simulink library "pne_pne3d_generic_std"  (R2016a)
settings: Solver=VariableStepAuto  StartTime=0.0  StopTime=10.0  RelTol=1e-3
undefined symbols (not defined in the file): sMP
(part 1 of 7)
settings Model: Creator=CAB  LastModifiedBy=CAB
settings GRTTargetCC: GeneratePreprocessorConditionals=Use local settings

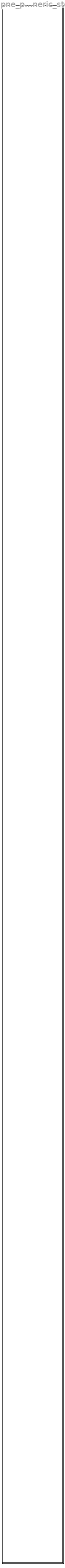
== system pne_pne3d_generic_std ==
  pne_pne3d_generic_std : Subsystem  mask{s1=sMP.phys.pne.settings_iMode, s2=sMP.phys.pne.settings_dt, initCmd='Parameters_pne_pne3d_generic_std_sf', p1=sMP.phys.pne.susp1.dxMax, p2=sMP.phys.pne.susp1.dxMin, p3=sMP.phys.pne.susp1.dxRef, p4=sMP.phys.pne.susp1.vLift, p5=sMP.phys.pne.susp1.vLow, p6=sMP.phys.pne.susp2.dxMax, p7=sMP.phys.pne.susp2.dxMin, p8=sMP.phys.pne.susp2.dxRef, p9=sMP.phys.pne.susp2.vLift, p10=sMP.phys.pne.susp2.vLow, p11=sMP.phys.pne.susp3.dxMax, p12=sMP.phys.pne.susp3.dxMin, p13=sMP.phys.pne.susp3.dxRef, p14=sMP.phys.pne.susp3.vLift, p15=sMP.phys.pne.susp3.vLow, p16=sMP.phys.pne.susp4.dxMax, p17=sMP.phys.pne.susp4.dxMin, p18=sMP.phys.pne.susp4.dxRef, p19=sMP.phys.pne.susp4.vLift, p20=sMP.phys.pne.susp4.vLow, p21=sMP.phys.pne.brk1.brakeType, p22=sMP.phys.pne.brk1.bt_A_norm, p23=sMP.phys.pne.brk1.bt_A_pad, p24=sMP.phys.pne.brk1.bt_alpha_conv_fac_cool, p25=sMP.phys.pne.brk1.bt_alpha_conv_fac_fric, p26=sMP.phys.pne.brk1.bt_base_conduction_corr, p27=sMP.phys.pne.brk1.bt_delta_r, p28=sMP.phys.pne.brk1.bt_density_correction, p29=sMP.phys.pne.brk1.bt_epsilon_corr, p30=sMP.phys.pne.brk1.bt_rad_offset, p31=sMP.phys.pne.brk1.bt_radiation_area_corr, p32=sMP.phys.pne.brk1.considerTg, p33=sMP.phys.pne.brk1.Cs, p34=sMP.phys.pne.brk1.eta, p35=sMP.phys.pne.brk1.fac_T_Dim, p36=sMP.phys.pne.brk1.fac_v_Dim, p37=sMP.phys.pne.brk1.Fdx_Dim, p38=sMP.phys.pne.brk1.Gwear, p39=sMP.phys.pne.brk1.i_Dim, p40=sMP.phys.pne.brk1.reff, p41=sMP.phys.pne.brk1.sPad_sum0, p42=sMP.phys.pne.brk1.useVarTempCalc, p43=sMP.phys.pne.brk1.wearRate_T_Dim, p44=sMP.phys.pne.brk2.brakeType, p45=sMP.phys.pne.brk2.bt_A_norm, p46=sMP.phys.pne.brk2.bt_A_pad, p47=sMP.phys.pne.brk2.bt_alpha_conv_fac_cool, p48=sMP.phys.pne.brk2.bt_alpha_conv_fac_fric, p49=sMP.phys.pne.brk2.bt_base_conduction_corr, p50=sMP.phys.pne.brk2.bt_delta_r, p51=sMP.phys.pne.brk2.bt_density_correction, p52=sMP.phys.pne.brk2.bt_epsilon_corr, p53=sMP.phys.pne.brk2.bt_rad_offset, p54=sMP.phys.pne.brk2.bt_radiation_area_corr, p55=sMP.phys.pne.brk2.considerTg, p56=sMP.phys.pne.brk2.Cs, p57=sMP.phys.pne.brk2.eta, p58=sMP.phys.pne.brk2.fac_T_Dim, p59=sMP.phys.pne.brk2.fac_v_Dim, p60=sMP.phys.pne.brk2.Fdx_Dim, p61=sMP.phys.pne.brk2.Gwear, p62=sMP.phys.pne.brk2.i_Dim, p63=sMP.phys.pne.brk2.reff, p64=sMP.phys.pne.brk2.sPad_sum0, p65=sMP.phys.pne.brk2.useVarTempCalc, p66=sMP.phys.pne.brk2.wearRate_T_Dim, p67=sMP.phys.pne.brk3.brakeType, p68=sMP.phys.pne.brk3.bt_A_norm, p69=sMP.phys.pne.brk3.bt_A_pad, p70=sMP.phys.pne.brk3.bt_alpha_conv_fac_cool, p71=sMP.phys.pne.brk3.bt_alpha_conv_fac_fric, p72=sMP.phys.pne.brk3.bt_base_conduction_corr, p73=sMP.phys.pne.brk3.bt_delta_r, p74=sMP.phys.pne.brk3.bt_density_correction, p75=sMP.phys.pne.brk3.bt_epsilon_corr, p76=sMP.phys.pne.brk3.bt_rad_offset, p77=sMP.phys.pne.brk3.bt_radiation_area_corr, p78=sMP.phys.pne.brk3.considerTg, p79=sMP.phys.pne.brk3.Cs, p80=sMP.phys.pne.brk3.eta, p81=sMP.phys.pne.brk3.fac_T_Dim, p82=sMP.phys.pne.brk3.fac_v_Dim, p83=sMP.phys.pne.brk3.Fdx_Dim, p84=sMP.phys.pne.brk3.Gwear, p85=sMP.phys.pne.brk3.i_Dim, p86=sMP.phys.pne.brk3.reff, p87=sMP.phys.pne.brk3.sPad_sum0, p88=sMP.phys.pne.brk3.useVarTempCalc, p89=sMP.phys.pne.brk3.wearRate_T_Dim, p90=sMP.phys.pne.brk4.brakeType, p91=sMP.phys.pne.brk4.bt_A_norm, p92=sMP.phys.pne.brk4.bt_A_pad, p93=sMP.phys.pne.brk4.bt_alpha_conv_fac_cool, p94=sMP.phys.pne.brk4.bt_alpha_conv_fac_fric, p95=sMP.phys.pne.brk4.bt_base_conduction_corr, p96=sMP.phys.pne.brk4.bt_delta_r, p97=sMP.phys.pne.brk4.bt_density_correction, p98=sMP.phys.pne.brk4.bt_epsilon_corr, p99=sMP.phys.pne.brk4.bt_rad_offset, p100=sMP.phys.pne.brk4.bt_radiation_area_corr, p101=sMP.phys.pne.brk4.considerTg, p102=sMP.phys.pne.brk4.Cs, p103=sMP.phys.pne.brk4.eta, p104=sMP.phys.pne.brk4.fac_T_Dim, p105=sMP.phys.pne.brk4.fac_v_Dim, p106=sMP.phys.pne.brk4.Fdx_Dim, p107=sMP.phys.pne.brk4.Gwear, p108=sMP.phys.pne.brk4.i_Dim, p109=sMP.phys.pne.brk4.reff, p110=sMP.phys.pne.brk4.sPad_sum0, p111=sMP.phys.pne.brk4.useVarTempCalc, p112=sMP.phys.pne.brk4.wearRate_T_Dim, p113=sMP.phys.pne.cyl1.dxFSpring_Dim, p114=sMP.phys.pne.cyl1.dxVolPB_Dim, p115=sMP.phys.pne.cyl1.dxVolSB_Dim, p116=sMP.phys.pne.cyl1.FNom, p117=sMP.phys.pne.cyl1.maxStroke, p118=sMP.phys.pne.cyl1.pApp, p119=sMP.phys.pne.cyl1.pNom, p120=sMP.phys.pne.cyl1.pR_PB, p121=sMP.phys.pne.cyl1.xR_PB, p122=sMP.phys.pne.cyl2.dxFSpring_Dim, p123=sMP.phys.pne.cyl2.dxVolPB_Dim, p124=sMP.phys.pne.cyl2.dxVolSB_Dim, p125=sMP.phys.pne.cyl2.FNom, p126=sMP.phys.pne.cyl2.maxStroke, p127=sMP.phys.pne.cyl2.pApp, p128=sMP.phys.pne.cyl2.pNom, p129=sMP.phys.pne.cyl2.pR_PB, p130=sMP.phys.pne.cyl2.xR_PB, p131=sMP.phys.pne.cyl3.dxFSpring_Dim, p132=sMP.phys.pne.cyl3.dxVolPB_Dim, p133=sMP.phys.pne.cyl3.dxVolSB_Dim, p134=sMP.phys.pne.cyl3.FNom, p135=sMP.phys.pne.cyl3.maxStroke, p136=sMP.phys.pne.cyl3.pApp, p137=sMP.phys.pne.cyl3.pNom, p138=sMP.phys.pne.cyl3.pR_PB, p139=sMP.phys.pne.cyl3.xR_PB, p140=sMP.phys.pne.cyl4.dxFSpring_Dim, p141=sMP.phys.pne.cyl4.dxVolPB_Dim, p142=sMP.phys.pne.cyl4.dxVolSB_Dim, p143=sMP.phys.pne.cyl4.FNom, p144=sMP.phys.pne.cyl4.maxStroke, p145=sMP.phys.pne.cyl4.pApp, p146=sMP.phys.pne.cyl4.pNom, p147=sMP.phys.pne.cyl4.pR_PB, p148=sMP.phys.pne.cyl4.xR_PB, p149=sMP.phys.pne.cylTrailer1.dxFSpring_Dim, p150=sMP.phys.pne.cylTrailer1.dxVolPB_Dim, p151=sMP.phys.pne.cylTrailer1.dxVolSB_Dim, p152=sMP.phys.pne.cylTrailer1.FNom, p153=sMP.phys.pne.cylTrailer1.maxStroke, p154=sMP.phys.pne.cylTrailer1.pApp, p155=sMP.phys.pne.cylTrailer1.pNom, p156=sMP.phys.pne.cylTrailer1.pR_PB, p157=sMP.phys.pne.cylTrailer1.xR_PB, p158=sMP.phys.pne.cylTrailer2.dxFSpring_Dim, p159=sMP.phys.pne.cylTrailer2.dxVolPB_Dim, p160=sMP.phys.pne.cylTrailer2.dxVolSB_Dim, p161=sMP.phys.pne.cylTrailer2.FNom, p162=sMP.phys.pne.cylTrailer2.maxStroke, p163=sMP.phys.pne.cylTrailer2.pApp, p164=sMP.phys.pne.cylTrailer2.pNom, p165=sMP.phys.pne.cylTrailer2.pR_PB, p166=sMP.phys.pne.cylTrailer2.xR_PB, p167=sMP.phys.pne.cylTrailer3.dxFSpring_Dim, p168=sMP.phys.pne.cylTrailer3.dxVolPB_Dim, p169=sMP.phys.pne.cylTrailer3.dxVolSB_Dim, p170=sMP.phys.pne.cylTrailer3.FNom, p171=sMP.phys.pne.cylTrailer3.maxStroke, p172=sMP.phys.pne.cylTrailer3.pApp, p173=sMP.phys.pne.cylTrailer3.pNom, p174=sMP.phys.pne.cylTrailer3.pR_PB, p175=sMP.phys.pne.cylTrailer3.xR_PB, p176=sMP.phys.pne.brkTrailer1.brakeType, p177=sMP.phys.pne.brkTrailer1.bt_A_norm, p178=sMP.phys.pne.brkTrailer1.bt_A_pad, p179=sMP.phys.pne.brkTrailer1.bt_alpha_conv_fac_cool, p180=sMP.phys.pne.brkTrailer1.bt_alpha_conv_fac_fric, p181=sMP.phys.pne.brkTrailer1.bt_base_conduction_corr, p182=sMP.phys.pne.brkTrailer1.bt_delta_r, p183=sMP.phys.pne.brkTrailer1.bt_density_correction, p184=sMP.phys.pne.brkTrailer1.bt_epsilon_corr, p185=sMP.phys.pne.brkTrailer1.bt_rad_offset, p186=sMP.phys.pne.brkTrailer1.bt_radiation_area_corr, p187=sMP.phys.pne.brkTrailer1.considerTg, p188=sMP.phys.pne.brkTrailer1.Cs, p189=sMP.phys.pne.brkTrailer1.eta, p190=sMP.phys.pne.brkTrailer1.fac_T_Dim, p191=sMP.phys.pne.brkTrailer1.fac_v_Dim, p192=sMP.phys.pne.brkTrailer1.Fdx_Dim, p193=sMP.phys.pne.brkTrailer1.Gwear, p194=sMP.phys.pne.brkTrailer1.i_Dim, p195=sMP.phys.pne.brkTrailer1.reff, p196=sMP.phys.pne.brkTrailer1.sPad_sum0, p197=sMP.phys.pne.brkTrailer1.useVarTempCalc, p198=sMP.phys.pne.brkTrailer1.wearRate_T_Dim, p199=sMP.phys.pne.brkTrailer2.brakeType, p200=sMP.phys.pne.brkTrailer2.bt_A_norm, p201=sMP.phys.pne.brkTrailer2.bt_A_pad, p202=sMP.phys.pne.brkTrailer2.bt_alpha_conv_fac_cool, p203=sMP.phys.pne.brkTrailer2.bt_alpha_conv_fac_fric, p204=sMP.phys.pne.brkTrailer2.bt_base_conduction_corr, p205=sMP.phys.pne.brkTrailer2.bt_delta_r, p206=sMP.phys.pne.brkTrailer2.bt_density_correction, p207=sMP.phys.pne.brkTrailer2.bt_epsilon_corr, p208=sMP.phys.pne.brkTrailer2.bt_rad_offset, p209=sMP.phys.pne.brkTrailer2.bt_radiation_area_corr, p210=sMP.phys.pne.brkTrailer2.considerTg, p211=sMP.phys.pne.brkTrailer2.Cs, p212=sMP.phys.pne.brkTrailer2.eta, p213=sMP.phys.pne.brkTrailer2.fac_T_Dim, p214=sMP.phys.pne.brkTrailer2.fac_v_Dim, p215=sMP.phys.pne.brkTrailer2.Fdx_Dim, p216=sMP.phys.pne.brkTrailer2.Gwear, p217=sMP.phys.pne.brkTrailer2.i_Dim, p218=sMP.phys.pne.brkTrailer2.reff, p219=sMP.phys.pne.brkTrailer2.sPad_sum0, p220=sMP.phys.pne.brkTrailer2.useVarTempCalc, p221=sMP.phys.pne.brkTrailer2.wearRate_T_Dim, p222=sMP.phys.pne.brkTrailer3.brakeType, p223=sMP.phys.pne.brkTrailer3.bt_A_norm, p224=sMP.phys.pne.brkTrailer3.bt_A_pad, p225=sMP.phys.pne.brkTrailer3.bt_alpha_conv_fac_cool, p226=sMP.phys.pne.brkTrailer3.bt_alpha_conv_fac_fric, p227=sMP.phys.pne.brkTrailer3.bt_base_conduction_corr, p228=sMP.phys.pne.brkTrailer3.bt_delta_r, p229=sMP.phys.pne.brkTrailer3.bt_density_correction, p230=sMP.phys.pne.brkTrailer3.bt_epsilon_corr, p231=sMP.phys.pne.brkTrailer3.bt_rad_offset, p232=sMP.phys.pne.brkTrailer3.bt_radiation_area_corr, p233=sMP.phys.pne.brkTrailer3.considerTg, p234=sMP.phys.pne.brkTrailer3.Cs, p235=sMP.phys.pne.brkTrailer3.eta, p236=sMP.phys.pne.brkTrailer3.fac_T_Dim, p237=sMP.phys.pne.brkTrailer3.fac_v_Dim, p238=sMP.phys.pne.brkTrailer3.Fdx_Dim, p239=sMP.phys.pne.brkTrailer3.Gwear, p240=sMP.phys.pne.brkTrailer3.i_Dim, p241=sMP.phys.pne.brkTrailer3.reff, p242=sMP.phys.pne.brkTrailer3.sPad_sum0, p243=sMP.phys.pne.brkTrailer3.useVarTempCalc, p244=sMP.phys.pne.brkTrailer3.wearRate_T_Dim, p245=sMP.phys.pne.circ.T_pipe_AM_ABSValve_FL, p246=sMP.phys.pne.circ.T_pipe_AM_ABSValve_FR, p247=sMP.phys.pne.circ.T_pipe_AM_BC_AL, p248=sMP.phys.pne.circ.T_pipe_AM_BC_AR, p249=sMP.phys.pne.circ.T_pipe_AM_BC_RL, p250=sMP.phys.pne.circ.T_pipe_AM_BC_RR, p251=sMP.phys.pne.circTrlr.flagTrailerABS, p252=sMP.phys.pne.circTrlr.T_pipe_Trailer_RV_Front, p253=sMP.phys.pne.circTrlr.T_pipe_Trailer_RV_Front_Rear, p254=sMP.phys.pne.circTrlr.VTrailer, p255=sMP.phys.pne.com.pACoverflow, p256=sMP.phys.pne.auxil.Drs_dVClose, p257=sMP.phys.pne.auxil.Drs_dVOpen, p258=sMP.phys.pne.auxil.Drs_pMeas, p259=sMP.phys.pne.auxil.Drs_tClose, p260=sMP.phys.pne.auxil.Drs_tOpen, p261=sMP.phys.pne.in.ebs_AdditionalAxle_left_pDmd, p262=sMP.phys.pne.in.ebs_AdditionalAxle_left_setABS, p263=sMP.phys.pne.in.ebs_AdditionalAxle_right_pDmd, p264=sMP.phys.pne.in.ebs_AdditionalAxle_right_setABS, p265=sMP.phys.pne.in.ebs_ESCsens_y_acceleration, p266=sMP.phys.pne.in.ebs_FrontAxle_left_pDmd, p267=sMP.phys.pne.in.ebs_FrontAxle_left_setABS, p268=sMP.phys.pne.in.ebs_FrontAxle_right_pDmd, p269=sMP.phys.pne.in.ebs_FrontAxle_right_setABS, p270=sMP.phys.pne.in.ebs_RearAxle_left_pDmd, p271=sMP.phys.pne.in.ebs_RearAxle_left_setABS, p272=sMP.phys.pne.in.ebs_RearAxle_right_pDmd, p273=sMP.phys.pne.in.ebs_RearAxle_right_setABS, p274=sMP.phys.pne.in.ebs_sBSP_stABSInValve_Addl_Left, p275=sMP.phys.pne.in.ebs_sBSP_stABSInValve_Addl_Right, p276=sMP.phys.pne.in.ebs_sBSP_stABSInValve_Front_Left, p277=sMP.phys.pne.in.ebs_sBSP_stABSInValve_Front_Right, p278=sMP.phys.pne.in.ebs_sBSP_stABSInValve_RCMax_Front, p279=sMP.phys.pne.in.ebs_sBSP_stABSInValve_RCMax_Rear, p280=sMP.phys.pne.in.ebs_sBSP_stABSInValve_Rear_Left, p281=sMP.phys.pne.in.ebs_sBSP_stABSInValve_Rear_Right, p282=sMP.phys.pne.in.ebs_sBSP_stABSOutValve_Addl_Left, p283=sMP.phys.pne.in.ebs_sBSP_stABSOutValve_Addl_Right, p284=sMP.phys.pne.in.ebs_sBSP_stABSOutValve_Front_Left, p285=sMP.phys.pne.in.ebs_sBSP_stABSOutValve_Front_Right, p286=sMP.phys.pne.in.ebs_sBSP_stABSOutValve_RCMax_Front, p287=sMP.phys.pne.in.ebs_sBSP_stABSOutValve_RCMax_Rear, p288=sMP.phys.pne.in.ebs_sBSP_stABSOutValve_Rear_Left, p289=sMP.phys.pne.in.ebs_sBSP_stABSOutValve_Rear_Right, p290=sMP.phys.pne.in.ebs_sBSP_stAPCVBuValve, p291=sMP.phys.pne.in.ebs_sBSP_stAPCVInValve, p292=sMP.phys.pne.in.ebs_sBSP_stAPCVOutValve, p293=sMP.phys.pne.in.ebs_sBSP_stAtcCutOffValve, p294=sMP.phys.pne.in.ebs_sBSP_stAxmoBuValve, p295=sMP.phys.pne.in.ebs_sBSP_stAxmoInValve_Rear_Left, p296=sMP.phys.pne.in.ebs_sBSP_stAxmoInValve_Rear_Right, p297=sMP.phys.pne.in.ebs_sBSP_stAxmoOutValve_Rear_Left, p298=sMP.phys.pne.in.ebs_sBSP_stAxmoOutValve_Rear_Right, p299=sMP.phys.pne.in.ebs_sBSP_stCMaxBuValve, p300=sMP.phys.pne.in.ebs_sBSP_stCMaxInValve_Rear_Left, p301=sMP.phys.pne.in.ebs_sBSP_stCMaxInValve_Rear_Right, p302=sMP.phys.pne.in.ebs_sBSP_stCMaxOutValve_Rear_Left, p303=sMP.phys.pne.in.ebs_sBSP_stCMaxOutValve_Rear_Right, p304=sMP.phys.pne.in.ebs_sBSP_stRCMaxInValve_Front, p305=sMP.phys.pne.in.ebs_sBSP_stRCMaxInValve_Rear, p306=sMP.phys.pne.in.ebs_sBSP_stRCMaxOutValve_Front, p307=sMP.phys.pne.in.ebs_sBSP_stRCMaxOutValve_Rear, p308=sMP.phys.pne.in.ebs_sBSP_stTCVBuValve, p309=sMP.phys.pne.in.ebs_sBSP_stTCVInValve, p310=sMP.phys.pne.in.ebs_sBSP_stTCVOutValve, p311=sMP.phys.pne.in.ebs_sil_AAle_force, p312=sMP.phys.pne.in.ebs_sil_AAle_vel, p313=sMP.phys.pne.in.ebs_sil_AAri_force, p314=sMP.phys.pne.in.ebs_sil_AAri_vel, p315=sMP.phys.pne.in.ebs_sil_FAle_force, p316=sMP.phys.pne.in.ebs_sil_FAle_vel, p317=sMP.phys.pne.in.ebs_sil_FAri_force, p318=sMP.phys.pne.in.ebs_sil_FAri_vel, p319=sMP.phys.pne.in.ebs_sil_RAle_force, p320=sMP.phys.pne.in.ebs_sil_RAle_vel, p321=sMP.phys.pne.in.ebs_sil_RAri_force, p322=sMP.phys.pne.in.ebs_sil_RAri_vel, p323=sMP.phys.pne.in.ebs_st3by2_First, p324=sMP.phys.pne.in.ebs_st3by2_Second, p325=sMP.phys.pne.in.ebs_TCV_pDmd, p326=sMP.phys.pne.in.env_air_frontVel, p327=sMP.phys.pne.in.env_pressure, p328=sMP.phys.pne.in.env_Temperature, p329=sMP.phys.pne.in.Failure_electric_circuit_AA, p330=sMP.phys.pne.in.Failure_electric_circuit_FA, p331=sMP.phys.pne.in.Failure_electric_circuit_RA, p332=sMP.phys.pne.in.Failure_pneumatic_circuit_FA, p333=sMP.phys.pne.in.Failure_pneumatic_circuit_RA, p334=sMP.phys.pne.out.pne_AirConsumptionFlow_AirSuspension, p335=sMP.phys.pne.out.pne_AirConsumptionFlow_auxiliaries, p336=sMP.phys.pne.out.pne_AirConsumptionFlow_doors, p337=sMP.phys.pne.out.pne_AirConsumptionFlow_EnduranceBrakes, p338=sMP.phys.pne.out.pne_AirConsumptionFlow_engine, p339=sMP.phys.pne.out.pne_AirConsumptionFlow_gearbox, p340=sMP.phys.pne.out.pne_AirConsumptionFlow_leakage, p341=sMP.phys.pne.out.pne_AirConsumptionFlow_PowerBoost, p342=sMP.phys.pne.out.pne_AirConsumptionFlow_SCR, p343=sMP.phys.pne.out.pne_brk_Actual_Pressure_AL, p344=sMP.phys.pne.out.pne_brk_Actual_Pressure_AR, p345=sMP.phys.pne.out.pne_brk_Actual_Pressure_FA, p346=sMP.phys.pne.out.pne_brk_Actual_Pressure_FOPB, p347=sMP.phys.pne.out.pne_brk_Actual_Pressure_Front, p348=sMP.phys.pne.out.pne_brk_Actual_Pressure_Rear, p349=sMP.phys.pne.out.pne_brk_Actual_Pressure_RL, p350=sMP.phys.pne.out.pne_brk_Actual_Pressure_RR, p351=sMP.phys.pne.out.pne_brk_Actual_Pressure_TCV, p352=sMP.phys.pne.out.pne_brk_AdditionalAxle_AxMo_left_rotVel, p353=sMP.phys.pne.out.pne_brk_AdditionalAxle_AxMo_right_rotVel, p354=sMP.phys.pne.out.pne_brk_AdditionalAxle_left_pAct, p355=sMP.phys.pne.out.pne_brk_AdditionalAxle_left_rotVel, p356=sMP.phys.pne.out.pne_brk_AdditionalAxle_right_pAct, p357=sMP.phys.pne.out.pne_brk_AdditionalAxle_right_rotVel, p358=sMP.phys.pne.in.pne_brk_AirCompressor_angAcc, p359=sMP.phys.pne.in.pne_brk_AirCompressor_angPos, p360=sMP.phys.pne.in.pne_brk_AirCompressor_angVel, p361=sMP.phys.pne.out.pne_brk_AirCompressor_delivery, p362=sMP.phys.pne.out.pne_brk_AirCompressor_torque, p363=sMP.phys.pne.out.pne_brk_AirConsumpEng_massfracH2O, p364=sMP.phys.pne.in.pne_brk_AirConsumpEng_mdot, p365=sMP.phys.pne.out.pne_brk_AirConsumpEng_pressure, p366=sMP.phys.pne.out.pne_brk_AirConsumpEng_Temperature, p367=sMP.phys.pne.out.pne_brk_AirConsumpRet_massfracH2O, p368=sMP.phys.pne.in.pne_brk_AirConsumpRet_mdot, p369=sMP.phys.pne.out.pne_brk_AirConsumpRet_pressure, p370=sMP.phys.pne.out.pne_brk_AirConsumpRet_Temperature, p371=sMP.phys.pne.out.pne_brk_AirConsumpTx_massfracH2O, p372=sMP.phys.pne.in.pne_brk_AirConsumpTx_mdot, p373=sMP.phys.pne.out.pne_brk_AirConsumpTx_pressure, p374=sMP.phys.pne.out.pne_brk_AirConsumpTx_Temperature, p375=sMP.phys.pne.out.pne_brk_Axle1_BrakingForce_at8p5bar, p376=sMP.phys.pne.out.pne_brk_Axle1_BrakingPower, p377=sMP.phys.pne.in.pne_brk_Axle1_left_angAcc, p378=sMP.phys.pne.in.pne_brk_Axle1_left_angPos, p379=sMP.phys.pne.in.pne_brk_Axle1_left_angVel, p380=sMP.phys.pne.out.pne_brk_Axle1_left_kvT, p381=sMP.phys.pne.out.pne_brk_Axle1_left_sPad_sum, p382=sMP.phys.pne.out.pne_brk_Axle1_left_Tcooldown, p383=sMP.phys.pne.out.pne_brk_Axle1_left_Tfriction, p384=sMP.phys.pne.out.pne_brk_Axle1_left_Tinterior, p385=sMP.phys.pne.out.pne_brk_Axle1_left_torque, p386=sMP.phys.pne.out.pne_brk_Axle1_left_torque_grinding, p387=sMP.phys.pne.in.pne_brk_Axle1_right_angAcc, p388=sMP.phys.pne.in.pne_brk_Axle1_right_angPos, p389=sMP.phys.pne.in.pne_brk_Axle1_right_angVel, p390=sMP.phys.pne.out.pne_brk_Axle1_right_kvT, p391=sMP.phys.pne.out.pne_brk_Axle1_right_sPad_sum, p392=sMP.phys.pne.out.pne_brk_Axle1_right_Tcooldown, p393=sMP.phys.pne.out.pne_brk_Axle1_right_Tfriction, p394=sMP.phys.pne.out.pne_brk_Axle1_right_Tinterior, p395=sMP.phys.pne.out.pne_brk_Axle1_right_torque, p396=sMP.phys.pne.out.pne_brk_Axle1_right_torque_grinding, p397=sMP.phys.pne.out.pne_brk_Axle1_torque_sns, p398=sMP.phys.pne.out.pne_brk_Axle1Brake_Fcyl, p399=sMP.phys.pne.out.pne_brk_Axle1Brake_left_pRel, p400=sMP.phys.pne.out.pne_brk_Axle1Brake_right_pRel, p401=sMP.phys.pne.out.pne_brk_Axle1Brake_stroke, p402=sMP.phys.pne.out.pne_brk_Axle1Brake_Vol, p403=sMP.phys.pne.out.pne_brk_Axle2_BrakingForce_at8p5bar, p404=sMP.phys.pne.out.pne_brk_Axle2_BrakingPower, p405=sMP.phys.pne.in.pne_brk_Axle2_left_angAcc, p406=sMP.phys.pne.in.pne_brk_Axle2_left_angPos, p407=sMP.phys.pne.in.pne_brk_Axle2_left_angVel, p408=sMP.phys.pne.out.pne_brk_Axle2_left_kvT, p409=sMP.phys.pne.out.pne_brk_Axle2_left_sPad_sum, p410=sMP.phys.pne.out.pne_brk_Axle2_left_Tcooldown, p411=sMP.phys.pne.out.pne_brk_Axle2_left_Tfriction, p412=sMP.phys.pne.out.pne_brk_Axle2_left_Tinterior, p413=sMP.phys.pne.out.pne_brk_Axle2_left_torque, p414=sMP.phys.pne.out.pne_brk_Axle2_left_torque_grinding, p415=sMP.phys.pne.in.pne_brk_Axle2_right_angAcc, p416=sMP.phys.pne.in.pne_brk_Axle2_right_angPos, p417=sMP.phys.pne.in.pne_brk_Axle2_right_angVel, p418=sMP.phys.pne.out.pne_brk_Axle2_right_kvT, p419=sMP.phys.pne.out.pne_brk_Axle2_right_sPad_sum, p420=sMP.phys.pne.out.pne_brk_Axle2_right_Tcooldown, p421=sMP.phys.pne.out.pne_brk_Axle2_right_Tfriction, p422=sMP.phys.pne.out.pne_brk_Axle2_right_Tinterior, p423=sMP.phys.pne.out.pne_brk_Axle2_right_torque, p424=sMP.phys.pne.out.pne_brk_Axle2_right_torque_grinding, p425=sMP.phys.pne.out.pne_brk_Axle2_torque_sns, p426=sMP.phys.pne.out.pne_brk_Axle2Brake_Fcyl, p427=sMP.phys.pne.out.pne_brk_Axle2Brake_left_pRel, p428=sMP.phys.pne.out.pne_brk_Axle2Brake_right_pRel, p429=sMP.phys.pne.out.pne_brk_Axle2Brake_stroke, p430=sMP.phys.pne.out.pne_brk_Axle2Brake_Vol, p431=sMP.phys.pne.out.pne_brk_Axle3_BrakingForce_at8p5bar, p432=sMP.phys.pne.out.pne_brk_Axle3_BrakingPower, p433=sMP.phys.pne.in.pne_brk_Axle3_left_angAcc, p434=sMP.phys.pne.in.pne_brk_Axle3_left_angPos, p435=sMP.phys.pne.in.pne_brk_Axle3_left_angVel, p436=sMP.phys.pne.out.pne_brk_Axle3_left_kvT, p437=sMP.phys.pne.out.pne_brk_Axle3_left_sPad_sum, p438=sMP.phys.pne.out.pne_brk_Axle3_left_Tcooldown, p439=sMP.phys.pne.out.pne_brk_Axle3_left_Tfriction, p440=sMP.phys.pne.out.pne_brk_Axle3_left_Tinterior, p441=sMP.phys.pne.out.pne_brk_Axle3_left_torque, p442=sMP.phys.pne.out.pne_brk_Axle3_left_torque_grinding, p443=sMP.phys.pne.in.pne_brk_Axle3_right_angAcc, p444=sMP.phys.pne.in.pne_brk_Axle3_right_angPos, p445=sMP.phys.pne.in.pne_brk_Axle3_right_angVel, p446=sMP.phys.pne.out.pne_brk_Axle3_right_kvT, p447=sMP.phys.pne.out.pne_brk_Axle3_right_sPad_sum, p448=sMP.phys.pne.out.pne_brk_Axle3_right_Tcooldown, p449=sMP.phys.pne.out.pne_brk_Axle3_right_Tfriction, p450=sMP.phys.pne.out.pne_brk_Axle3_right_Tinterior, p451=sMP.phys.pne.out.pne_brk_Axle3_right_torque, p452=sMP.phys.pne.out.pne_brk_Axle3_right_torque_grinding, p453=sMP.phys.pne.out.pne_brk_Axle3_torque_sns, p454=sMP.phys.pne.out.pne_brk_Axle3Brake_Fcyl, p455=sMP.phys.pne.out.pne_brk_Axle3Brake_left_pRel, p456=sMP.phys.pne.out.pne_brk_Axle3Brake_right_pRel, p457=sMP.phys.pne.out.pne_brk_Axle3Brake_stroke, p458=sMP.phys.pne.out.pne_brk_Axle3Brake_Vol, p459=sMP.phys.pne.out.pne_brk_Axle4_BrakingForce_at8p5bar, p460=sMP.phys.pne.out.pne_brk_Axle4_BrakingPower, p461=sMP.phys.pne.in.pne_brk_Axle4_left_angAcc, p462=sMP.phys.pne.in.pne_brk_Axle4_left_angPos, p463=sMP.phys.pne.in.pne_brk_Axle4_left_angVel, p464=sMP.phys.pne.out.pne_brk_Axle4_left_kvT, p465=sMP.phys.pne.out.pne_brk_Axle4_left_sPad_sum, p466=sMP.phys.pne.out.pne_brk_Axle4_left_Tcooldown, p467=sMP.phys.pne.out.pne_brk_Axle4_left_Tfriction, p468=sMP.phys.pne.out.pne_brk_Axle4_left_Tinterior, p469=sMP.phys.pne.out.pne_brk_Axle4_left_torque, p470=sMP.phys.pne.out.pne_brk_Axle4_left_torque_grinding, p471=sMP.phys.pne.in.pne_brk_Axle4_right_angAcc, p472=sMP.phys.pne.in.pne_brk_Axle4_right_angPos, p473=sMP.phys.pne.in.pne_brk_Axle4_right_angVel, p474=sMP.phys.pne.out.pne_brk_Axle4_right_kvT, p475=sMP.phys.pne.out.pne_brk_Axle4_right_sPad_sum, p476=sMP.phys.pne.out.pne_brk_Axle4_right_Tcooldown, p477=sMP.phys.pne.out.pne_brk_Axle4_right_Tfriction, p478=sMP.phys.pne.out.pne_brk_Axle4_right_Tinterior, p479=sMP.phys.pne.out.pne_brk_Axle4_right_torque, p480=sMP.phys.pne.out.pne_brk_Axle4_right_torque_grinding, p481=sMP.phys.pne.out.pne_brk_Axle4_torque_sns, p482=sMP.phys.pne.out.pne_brk_Axle4Brake_Fcyl, p483=sMP.phys.pne.out.pne_brk_Axle4Brake_left_pRel, p484=sMP.phys.pne.out.pne_brk_Axle4Brake_right_pRel, p485=sMP.phys.pne.out.pne_brk_Axle4Brake_stroke, p486=sMP.phys.pne.out.pne_brk_Axle4Brake_Vol, p487=sMP.phys.pne.out.pne_brk_BrkWearAALt, p488=sMP.phys.pne.out.pne_brk_BrkWearAARt, p489=sMP.phys.pne.out.pne_brk_BrkWearFA1Lt, p490=sMP.phys.pne.out.pne_brk_BrkWearFA1Rt, p491=sMP.phys.pne.out.pne_brk_BrkWearFA2Lt, p492=sMP.phys.pne.out.pne_brk_BrkWearFA2Rt, p493=sMP.phys.pne.out.pne_brk_BrkWearRA1Lt, p494=sMP.phys.pne.out.pne_brk_BrkWearRA1Rt, p495=sMP.phys.pne.out.pne_brk_BrkWearRA2Lt, p496=sMP.phys.pne.out.pne_brk_BrkWearRA2Rt, p497=sMP.phys.pne.out.pne_brk_CompON, p498=sMP.phys.pne.out.pne_brk_CompOut_Temp, p499=sMP.phys.pne.in.pne_brk_CompressorInlet_massfracH2O, p500=sMP.phys.pne.out.pne_brk_CompressorInlet_mdot, p501=sMP.phys.pne.in.pne_brk_CompressorInlet_pressure, p502=sMP.phys.pne.in.pne_brk_CompressorInlet_Temperature, p503=sMP.phys.pne.out.pne_brk_CoolingPipe_pRel, p504=sMP.phys.pne.out.pne_brk_CoolingPipe_Temp, p505=sMP.phys.pne.out.pne_brk_EAPU_pRel, p506=sMP.phys.pne.out.pne_brk_EAPU_Temp, p507=sMP.phys.pne.out.pne_brk_FrontAxle_left_rotVel, p508=sMP.phys.pne.out.pne_brk_FrontAxle_pAct, p509=sMP.phys.pne.out.pne_brk_FrontAxle_right_rotVel, p510=sMP.phys.pne.out.pne_brk_PowerBoost_massfracH2O, p511=sMP.phys.pne.in.pne_brk_PowerBoost_mdot, p512=sMP.phys.pne.out.pne_brk_PowerBoost_pressure, p513=sMP.phys.pne.out.pne_brk_PowerBoost_Temperature, p514=sMP.phys.pne.out.pne_brk_pRelPkBrk, p515=sMP.phys.pne.out.pne_brk_RearAxle_left_pAct, p516=sMP.phys.pne.out.pne_brk_RearAxle_left_rotVel, p517=sMP.phys.pne.out.pne_brk_RearAxle_right_pAct, p518=sMP.phys.pne.out.pne_brk_RearAxle_right_rotVel, p519=sMP.phys.pne.out.pne_brk_reg_active, p520=sMP.phys.pne.out.pne_brk_rotVel_al, p521=sMP.phys.pne.out.pne_brk_rotVel_ar, p522=sMP.phys.pne.out.pne_brk_rotVel_fl, p523=sMP.phys.pne.out.pne_brk_rotVel_fr, p524=sMP.phys.pne.out.pne_brk_rotVel_rl, p525=sMP.phys.pne.out.pne_brk_rotVel_rr, p526=sMP.phys.pne.out.pne_brk_rotVel_t1l, p527=sMP.phys.pne.out.pne_brk_rotVel_t1r, p528=sMP.phys.pne.out.pne_brk_rotVel_t2l, p529=sMP.phys.pne.out.pne_brk_rotVel_t2r, p530=sMP.phys.pne.out.pne_brk_rotVel_t3l, p531=sMP.phys.pne.out.pne_brk_rotVel_t3r, p532=sMP.phys.pne.out.pne_brk_TCV_pAct, p533=sMP.phys.pne.out.pne_brk_Trailer_RV_Front_pAct, p534=sMP.phys.pne.out.pne_brk_Trailer_RV_Rear_pAct, p535=sMP.phys.pne.out.pne_brk_TrailerAxle1_BrakingForce_at8p5bar, p536=sMP.phys.pne.out.pne_brk_TrailerAxle1_BrakingPower, p537=sMP.phys.pne.in.pne_brk_TrailerAxle1_left_angAcc, p538=sMP.phys.pne.in.pne_brk_TrailerAxle1_left_angPos, p539=sMP.phys.pne.in.pne_brk_TrailerAxle1_left_angVel, p540=sMP.phys.pne.out.pne_brk_TrailerAxle1_left_kvT, p541=sMP.phys.pne.out.pne_brk_TrailerAxle1_left_sPad_sum, p542=sMP.phys.pne.out.pne_brk_TrailerAxle1_left_Tcooldown, p543=sMP.phys.pne.out.pne_brk_TrailerAxle1_left_Tfriction, p544=sMP.phys.pne.out.pne_brk_TrailerAxle1_left_Tinterior, p545=sMP.phys.pne.out.pne_brk_TrailerAxle1_left_torque, p546=sMP.phys.pne.out.pne_brk_TrailerAxle1_left_torque_grinding, p547=sMP.phys.pne.in.pne_brk_TrailerAxle1_right_angAcc, p548=sMP.phys.pne.in.pne_brk_TrailerAxle1_right_angPos, p549=sMP.phys.pne.in.pne_brk_TrailerAxle1_right_angVel, p550=sMP.phys.pne.out.pne_brk_TrailerAxle1_right_kvT, p551=sMP.phys.pne.out.pne_brk_TrailerAxle1_right_sPad_sum, p552=sMP.phys.pne.out.pne_brk_TrailerAxle1_right_Tcooldown, p553=sMP.phys.pne.out.pne_brk_TrailerAxle1_right_Tfriction, p554=sMP.phys.pne.out.pne_brk_TrailerAxle1_right_Tinterior, p555=sMP.phys.pne.out.pne_brk_TrailerAxle1_right_torque, p556=sMP.phys.pne.out.pne_brk_TrailerAxle1_right_torque_grinding, p557=sMP.phys.pne.out.pne_brk_TrailerAxle1_torque_sns, p558=sMP.phys.pne.out.pne_brk_TrailerAxle1Brake_Fcyl, p559=sMP.phys.pne.out.pne_brk_TrailerAxle1Brake_left_pRel, p560=sMP.phys.pne.out.pne_brk_TrailerAxle1Brake_right_pRel, p561=sMP.phys.pne.out.pne_brk_TrailerAxle1Brake_stroke, p562=sMP.phys.pne.out.pne_brk_TrailerAxle1Brake_Vol, p563=sMP.phys.pne.out.pne_brk_TrailerAxle2_BrakingForce_at8p5bar, p564=sMP.phys.pne.out.pne_brk_TrailerAxle2_BrakingPower, p565=sMP.phys.pne.in.pne_brk_TrailerAxle2_left_angAcc, p566=sMP.phys.pne.in.pne_brk_TrailerAxle2_left_angPos, p567=sMP.phys.pne.in.pne_brk_TrailerAxle2_left_angVel, p568=sMP.phys.pne.out.pne_brk_TrailerAxle2_left_kvT, p569=sMP.phys.pne.out.pne_brk_TrailerAxle2_left_sPad_sum, p570=sMP.phys.pne.out.pne_brk_TrailerAxle2_left_Tcooldown, p571=sMP.phys.pne.out.pne_brk_TrailerAxle2_left_Tfriction, p572=sMP.phys.pne.out.pne_brk_TrailerAxle2_left_Tinterior, p573=sMP.phys.pne.out.pne_brk_TrailerAxle2_left_torque, p574=sMP.phys.pne.out.pne_brk_TrailerAxle2_left_torque_grinding, p575=sMP.phys.pne.in.pne_brk_TrailerAxle2_right_angAcc, p576=sMP.phys.pne.in.pne_brk_TrailerAxle2_right_angPos, p577=sMP.phys.pne.in.pne_brk_TrailerAxle2_right_angVel, p578=sMP.phys.pne.out.pne_brk_TrailerAxle2_right_kvT, p579=sMP.phys.pne.out.pne_brk_TrailerAxle2_right_sPad_sum, p580=sMP.phys.pne.out.pne_brk_TrailerAxle2_right_Tcooldown, p581=sMP.phys.pne.out.pne_brk_TrailerAxle2_right_Tfriction, p582=sMP.phys.pne.out.pne_brk_TrailerAxle2_right_Tinterior, p583=sMP.phys.pne.out.pne_brk_TrailerAxle2_right_torque, p584=sMP.phys.pne.out.pne_brk_TrailerAxle2_right_torque_grinding, p585=sMP.phys.pne.out.pne_brk_TrailerAxle2_torque_sns, p586=sMP.phys.pne.out.pne_brk_TrailerAxle2Brake_Fcyl, p587=sMP.phys.pne.out.pne_brk_TrailerAxle2Brake_left_pRel, p588=sMP.phys.pne.out.pne_brk_TrailerAxle2Brake_right_pRel, p589=sMP.phys.pne.out.pne_brk_TrailerAxle2Brake_stroke, p590=sMP.phys.pne.out.pne_brk_TrailerAxle2Brake_Vol, p591=sMP.phys.pne.out.pne_brk_TrailerAxle3_BrakingForce_at8p5bar, p592=sMP.phys.pne.out.pne_brk_TrailerAxle3_BrakingPower, p593=sMP.phys.pne.in.pne_brk_TrailerAxle3_left_angAcc, p594=sMP.phys.pne.in.pne_brk_TrailerAxle3_left_angPos, p595=sMP.phys.pne.in.pne_brk_TrailerAxle3_left_angVel, p596=sMP.phys.pne.out.pne_brk_TrailerAxle3_left_kvT, p597=sMP.phys.pne.out.pne_brk_TrailerAxle3_left_sPad_sum, p598=sMP.phys.pne.out.pne_brk_TrailerAxle3_left_Tcooldown, p599=sMP.phys.pne.out.pne_brk_TrailerAxle3_left_Tfriction, p600=sMP.phys.pne.out.pne_brk_TrailerAxle3_left_Tinterior, p601=sMP.phys.pne.out.pne_brk_TrailerAxle3_left_torque, p602=sMP.phys.pne.out.pne_brk_TrailerAxle3_left_torque_grinding, p603=sMP.phys.pne.in.pne_brk_TrailerAxle3_right_angAcc, p604=sMP.phys.pne.in.pne_brk_TrailerAxle3_right_angPos, p605=sMP.phys.pne.in.pne_brk_TrailerAxle3_right_angVel, p606=sMP.phys.pne.out.pne_brk_TrailerAxle3_right_kvT, p607=sMP.phys.pne.out.pne_brk_TrailerAxle3_right_sPad_sum, p608=sMP.phys.pne.out.pne_brk_TrailerAxle3_right_Tcooldown, p609=sMP.phys.pne.out.pne_brk_TrailerAxle3_right_Tfriction, p610=sMP.phys.pne.out.pne_brk_TrailerAxle3_right_Tinterior, p611=sMP.phys.pne.out.pne_brk_TrailerAxle3_right_torque, p612=sMP.phys.pne.out.pne_brk_TrailerAxle3_right_torque_grinding, p613=sMP.phys.pne.out.pne_brk_TrailerAxle3_torque_sns, p614=sMP.phys.pne.out.pne_brk_TrailerAxle3Brake_Fcyl, p615=sMP.phys.pne.out.pne_brk_TrailerAxle3Brake_left_pRel, p616=sMP.phys.pne.out.pne_brk_TrailerAxle3Brake_right_pRel, p617=sMP.phys.pne.out.pne_brk_TrailerAxle3Brake_stroke, p618=sMP.phys.pne.out.pne_brk_TrailerAxle3Brake_Vol, p619=sMP.phys.pne.out.pne_brk_V1_pRel, p620=sMP.phys.pne.out.pne_brk_V1_Temp, p621=sMP.phys.pne.out.pne_brk_V2_pRel, p622=sMP.phys.pne.out.pne_brk_V2_Temp, p623=sMP.phys.pne.out.pne_brk_V3_pRel, p624=sMP.phys.pne.out.pne_brk_V3_Temp, p625=sMP.phys.pne.out.pne_brk_V4_pRel, p626=sMP.phys.pne.out.pne_brk_V4_Temp, p627=sMP.phys.pne.out.pne_brk_V5_pRel, p628=sMP.phys.pne.out.pne_brk_V5_Temp, p629=sMP.phys.pne.out.pne_brk_V6_pRel, p630=sMP.phys.pne.out.pne_brk_V6_Temp, p631=sMP.phys.pne.out.pne_brk_V7_pRel, p632=sMP.phys.pne.out.pne_brk_V7_Temp, p633=sMP.phys.pne.out.pne_brk_V8_pRel, p634=sMP.phys.pne.out.pne_brk_V8_Temp, p635=sMP.phys.pne.out.pne_brk_Vsup_pRel, p636=sMP.phys.pne.out.pne_brk_Vsup_Temp, p637=sMP.phys.pne.out.pne_brk_VTrailer_pRel, p638=sMP.phys.pne.out.pne_brk_VTrailer_Temp, p639=sMP.phys.pne.out.pne_brk_WetLvl_Cntr, p640=sMP.phys.pne.out.pne_susp_A1_Le_Posn, p641=sMP.phys.pne.out.pne_susp_A1_Ri_Posn, p642=sMP.phys.pne.out.pne_susp_A2_Le_Posn, p643=sMP.phys.pne.out.pne_susp_A2_Ri_Posn, p644=sMP.phys.pne.out.pne_susp_A3_Le_Posn, p645=sMP.phys.pne.out.pne_susp_A3_Ri_Posn, p646=sMP.phys.pne.in.pneAux_A1_Le_Rq, p647=sMP.phys.pne.in.pneAux_A1_LoLi_Rq, p648=sMP.phys.pne.in.pneAux_A1_Ri_Rq, p649=sMP.phys.pne.in.pneAux_A2_Le_Rq, p650=sMP.phys.pne.in.pneAux_A2_LoLi_Rq, p651=sMP.phys.pne.in.pneAux_A2_Ri_Rq, p652=sMP.phys.pne.in.pneAux_A3_Le_Rq, p653=sMP.phys.pne.in.pneAux_A3_LoLi_Rq, p654=sMP.phys.pne.in.pneAux_A3_Ri_Rq, p655=sMP.phys.pne.in.pneAux_Axle1_load, p656=sMP.phys.pne.in.pneAux_Axle2_load, p657=sMP.phys.pne.in.pneAux_Axle3_load, p658=sMP.phys.pne.in.pneAux_Axle4_load, p659=sMP.phys.pne.in.pneAux_Drs_Rq, p660=sMP.phys.pne.in.pneAux_EAPU_overrun, p661=sMP.phys.pne.in.pneAux_pSoll_TCV_p43, p662=sMP.phys.pne.in.pneAux_pSollPkBrk, p663=sMP.phys.pne.in.pneAux_TCV_pDmd_Front_Left, p664=sMP.phys.pne.in.pneAux_TCV_pDmd_Front_Right, p665=sMP.phys.pne.in.pneAux_TCV_pDmd_Rear_Left, p666=sMP.phys.pne.in.pneAux_TCV_pDmd_Rear_Right, p667=sMP.phys.pne.in.pneAux_trailerAxle1_left_stABSInValve, p668=sMP.phys.pne.in.pneAux_trailerAxle1_left_stABSOutValve, p669=sMP.phys.pne.in.pneAux_trailerAxle1_load, p670=sMP.phys.pne.in.pneAux_trailerAxle1_right_stABSInValve, p671=sMP.phys.pne.in.pneAux_trailerAxle1_right_stABSOutValve, p672=sMP.phys.pne.in.pneAux_trailerAxle2_left_stABSInValve, p673=sMP.phys.pne.in.pneAux_trailerAxle2_left_stABSOutValve, p674=sMP.phys.pne.in.pneAux_trailerAxle2_load, p675=sMP.phys.pne.in.pneAux_trailerAxle2_right_stABSInValve, p676=sMP.phys.pne.in.pneAux_trailerAxle2_right_stABSOutValve, p677=sMP.phys.pne.in.pneAux_trailerAxle3_left_stABSInValve, p678=sMP.phys.pne.in.pneAux_trailerAxle3_left_stABSOutValve, p679=sMP.phys.pne.in.pneAux_trailerAxle3_load, p680=sMP.phys.pne.in.pneAux_trailerAxle3_right_stABSInValve, p681=sMP.phys.pne.in.pneAux_trailerAxle3_right_stABSOutValve, p682=sMP.phys.pne.auxil.QnLeak, p683=sMP.phys.pne.veh.stepSize, p684=sMP.phys.pne.veh.T1_APCV, p685=sMP.phys.pne.veh.T1_CMAX, p686=sMP.phys.pne.pro.dT_CompInlet, p687=sMP.phys.pne.pro.flagUS, p688=sMP.phys.pne.pro.pRelCI, p689=sMP.phys.pne.pro.pRelCI_RO, p690=sMP.phys.pne.pro.pRelCO, p691=sMP.phys.pne.pro.pRelCO_RO, p692=sMP.phys.pne.pro.pRelLimit_C1C2, p693=sMP.phys.pne.pro.pRelLimit_C3C4, p694=sMP.phys.pne.pro.RegenPct, p695=sMP.phys.pne.pro.V1, p696=sMP.phys.pne.pro.V2, p697=sMP.phys.pne.pro.V3, p698=sMP.phys.pne.pro.V4, p699=sMP.phys.pne.pro.V5, p700=sMP.phys.pne.pro.V6, p701=sMP.phys.pne.pro.V7, p702=sMP.phys.pne.pro.V8, p703=sMP.phys.pne.pro.Vcartridge, p704=sMP.phys.pne.pro.Vintake, p705=sMP.phys.pne.pro.Vreg, p706=sMP.phys.pne.pro.Vsup, p707=sMP.phys.pne.auxil.QnSCR, p708=sMP.phys.pne.initialTemperatures.TemperatureCalculation, p709=sMP.phys.pne.susp1.dV_mAxle_Ref, p710=sMP.phys.pne.susp2.dV_mAxle_Ref, p711=sMP.phys.pne.susp3.dV_mAxle_Ref, p712=sMP.phys.pne.susp4.dV_mAxle_Ref, p713=sMP.phys.pne.brk1.fac_T_xAxis, p714=sMP.phys.pne.brk1.fac_T_yAxis, p715=sMP.phys.pne.brk1.fac_v_xAxis, p716=sMP.phys.pne.brk1.fac_v_yAxis, p717=sMP.phys.pne.brk1.Fdx_xAxis, p718=sMP.phys.pne.brk1.Fdx_yAxis, p719=sMP.phys.pne.brk1.i_xAxis, p720=sMP.phys.pne.brk1.i_yAxis, p721=sMP.phys.pne.brk1.wearRate_T_xAxis, p722=sMP.phys.pne.brk1.wearRate_T_yAxis, p723=sMP.phys.pne.brk2.fac_T_xAxis, p724=sMP.phys.pne.brk2.fac_T_yAxis, p725=sMP.phys.pne.brk2.fac_v_xAxis, p726=sMP.phys.pne.brk2.fac_v_yAxis, p727=sMP.phys.pne.brk2.Fdx_xAxis, p728=sMP.phys.pne.brk2.Fdx_yAxis, p729=sMP.phys.pne.brk2.i_xAxis, p730=sMP.phys.pne.brk2.i_yAxis, p731=sMP.phys.pne.brk2.wearRate_T_xAxis, p732=sMP.phys.pne.brk2.wearRate_T_yAxis, p733=sMP.phys.pne.brk3.fac_T_xAxis, p734=sMP.phys.pne.brk3.fac_T_yAxis, p735=sMP.phys.pne.brk3.fac_v_xAxis, p736=sMP.phys.pne.brk3.fac_v_yAxis, p737=sMP.phys.pne.brk3.Fdx_xAxis, p738=sMP.phys.pne.brk3.Fdx_yAxis, p739=sMP.phys.pne.brk3.i_xAxis, p740=sMP.phys.pne.brk3.i_yAxis, p741=sMP.phys.pne.brk3.wearRate_T_xAxis, p742=sMP.phys.pne.brk3.wearRate_T_yAxis, p743=sMP.phys.pne.brk4.fac_T_xAxis, p744=sMP.phys.pne.brk4.fac_T_yAxis, p745=sMP.phys.pne.brk4.fac_v_xAxis, p746=sMP.phys.pne.brk4.fac_v_yAxis, p747=sMP.phys.pne.brk4.Fdx_xAxis, p748=sMP.phys.pne.brk4.Fdx_yAxis, p749=sMP.phys.pne.brk4.i_xAxis, p750=sMP.phys.pne.brk4.i_yAxis, p751=sMP.phys.pne.brk4.wearRate_T_xAxis, p752=sMP.phys.pne.brk4.wearRate_T_yAxis, p753=sMP.phys.pne.cyl1.dxFSpring_xAxis, p754=sMP.phys.pne.cyl1.dxFSpring_yAxis, p755=sMP.phys.pne.cyl1.dxVolPB_xAxis, p756=sMP.phys.pne.cyl1.dxVolPB_yAxis, p757=sMP.phys.pne.cyl1.dxVolSB_xAxis, p758=sMP.phys.pne.cyl1.dxVolSB_yAxis, p759=sMP.phys.pne.cyl2.dxFSpring_xAxis, p760=sMP.phys.pne.cyl2.dxFSpring_yAxis, p761=sMP.phys.pne.cyl2.dxVolPB_xAxis, p762=sMP.phys.pne.cyl2.dxVolPB_yAxis, p763=sMP.phys.pne.cyl2.dxVolSB_xAxis, p764=sMP.phys.pne.cyl2.dxVolSB_yAxis, p765=sMP.phys.pne.cyl3.dxFSpring_xAxis, p766=sMP.phys.pne.cyl3.dxFSpring_yAxis, p767=sMP.phys.pne.cyl3.dxVolPB_xAxis, p768=sMP.phys.pne.cyl3.dxVolPB_yAxis, p769=sMP.phys.pne.cyl3.dxVolSB_xAxis, p770=sMP.phys.pne.cyl3.dxVolSB_yAxis, p771=sMP.phys.pne.cyl4.dxFSpring_xAxis, p772=sMP.phys.pne.cyl4.dxFSpring_yAxis, p773=sMP.phys.pne.cyl4.dxVolPB_xAxis, p774=sMP.phys.pne.cyl4.dxVolPB_yAxis, p775=sMP.phys.pne.cyl4.dxVolSB_xAxis, p776=sMP.phys.pne.cyl4.dxVolSB_yAxis, p777=sMP.phys.pne.cylTrailer1.dxFSpring_xAxis, p778=sMP.phys.pne.cylTrailer1.dxFSpring_yAxis, p779=sMP.phys.pne.cylTrailer1.dxVolPB_xAxis, p780=sMP.phys.pne.cylTrailer1.dxVolPB_yAxis, p781=sMP.phys.pne.cylTrailer1.dxVolSB_xAxis, p782=sMP.phys.pne.cylTrailer1.dxVolSB_yAxis, p783=sMP.phys.pne.cylTrailer2.dxFSpring_xAxis, p784=sMP.phys.pne.cylTrailer2.dxFSpring_yAxis, p785=sMP.phys.pne.cylTrailer2.dxVolPB_xAxis, p786=sMP.phys.pne.cylTrailer2.dxVolPB_yAxis, p787=sMP.phys.pne.cylTrailer2.dxVolSB_xAxis, p788=sMP.phys.pne.cylTrailer2.dxVolSB_yAxis, p789=sMP.phys.pne.cylTrailer3.dxFSpring_xAxis, p790=sMP.phys.pne.cylTrailer3.dxFSpring_yAxis, p791=sMP.phys.pne.cylTrailer3.dxVolPB_xAxis, p792=sMP.phys.pne.cylTrailer3.dxVolPB_yAxis, p793=sMP.phys.pne.cylTrailer3.dxVolSB_xAxis, p794=sMP.phys.pne.cylTrailer3.dxVolSB_yAxis, p795=sMP.phys.pne.brkTrailer1.fac_T_xAxis, p796=sMP.phys.pne.brkTrailer1.fac_T_yAxis, p797=sMP.phys.pne.brkTrailer1.fac_v_xAxis, p798=sMP.phys.pne.brkTrailer1.fac_v_yAxis, p799=sMP.phys.pne.brkTrailer1.Fdx_xAxis, p800=sMP.phys.pne.brkTrailer1.Fdx_yAxis, p801=sMP.phys.pne.brkTrailer1.i_xAxis, p802=sMP.phys.pne.brkTrailer1.i_yAxis, p803=sMP.phys.pne.brkTrailer1.wearRate_T_xAxis, p804=sMP.phys.pne.brkTrailer1.wearRate_T_yAxis, p805=sMP.phys.pne.brkTrailer2.fac_T_xAxis, p806=sMP.phys.pne.brkTrailer2.fac_T_yAxis, p807=sMP.phys.pne.brkTrailer2.fac_v_xAxis, p808=sMP.phys.pne.brkTrailer2.fac_v_yAxis, p809=sMP.phys.pne.brkTrailer2.Fdx_xAxis, p810=sMP.phys.pne.brkTrailer2.Fdx_yAxis, p811=sMP.phys.pne.brkTrailer2.i_xAxis, p812=sMP.phys.pne.brkTrailer2.i_yAxis, p813=sMP.phys.pne.brkTrailer2.wearRate_T_xAxis, p814=sMP.phys.pne.brkTrailer2.wearRate_T_yAxis, p815=sMP.phys.pne.brkTrailer3.fac_T_xAxis, p816=sMP.phys.pne.brkTrailer3.fac_T_yAxis, p817=sMP.phys.pne.brkTrailer3.fac_v_xAxis, p818=sMP.phys.pne.brkTrailer3.fac_v_yAxis, p819=sMP.phys.pne.brkTrailer3.Fdx_xAxis, p820=sMP.phys.pne.brkTrailer3.Fdx_yAxis, p821=sMP.phys.pne.brkTrailer3.i_xAxis, p822=sMP.phys.pne.brkTrailer3.i_yAxis, p823=sMP.phys.pne.brkTrailer3.wearRate_T_xAxis, p824=sMP.phys.pne.brkTrailer3.wearRate_T_yAxis, p825=sMP.phys.pne.circ.brkCircuit, p826=sMP.phys.pne.circ.speedSensorPosnVeh, p827=sMP.phys.pne.circ.t_asymp75, p828=sMP.phys.pne.circ.t_release10, p829=sMP.phys.pne.circTrlr.brkCircuitTrailer, p830=sMP.phys.pne.circTrlr.flagTrailerControlActive, p831=sMP.phys.pne.circTrlr.speedSensorPosnTrailer, p832=sMP.phys.pne.circTrlr.t_asymp75_Trlr, p833=sMP.phys.pne.circTrlr.t_release10_Trlr, p834=sMP.phys.pne.com.dim_PmechMap, p835=sMP.phys.pne.com.dim_QnMap, p836=sMP.phys.pne.com.dim_ToutMap, p837=sMP.phys.pne.com.Pmech_Map_kW, p838=sMP.phys.pne.com.Pmech_x_om_rpm, p839=sMP.phys.pne.com.Pmech_y_dp_bar, p840=sMP.phys.pne.com.Qn_Map_l_min, p841=sMP.phys.pne.com.Qn_x_om_rpm, p842=sMP.phys.pne.com.Qn_y_dp_bar, p843=sMP.phys.pne.com.Tout_Map_degC, p844=sMP.phys.pne.com.Tout_x_om_rpm, p845=sMP.phys.pne.com.Tout_y_dp_bar, p846=sMP.phys.pne.veh.axleLoadTractor_kg, p847=sMP.phys.pne.veh.axleLoadTrailer_kg, p848=sMP.phys.pne.veh.AxleSpringType, p849=sMP.phys.pne.veh.pAppCyl_Tractor, p850=sMP.phys.pne.veh.pAppCyl_Trailer, p851=sMP.phys.pne.veh.rdynTractor, p852=sMP.phys.pne.veh.rdynTrailer, p853=sMP.phys.pne.veh.axleLoadTrailer02_kg, p854=sMP.phys.pne.veh.pAppCyl_Trailer02, p855=sMP.phys.pne.veh.rdynTrailer02, p856=sMP.phys.pne.initialTemperatures.initial_wear, p857=sMP.phys.pne.initialTemperatures.T_initial_brakes}
